simulink model "LQI_controller"  (R2024b)
settings: Solver=VariableStepAuto  StartTime=0.0  StopTime=10  RelTol=1e-3
values from neighbouring files (symbols this model uses):
  K = -F(1:2)    [State_Space_Controller.m]
  N = -F(3)    [State_Space_Controller.m]
  Ts = 0.01    [Controller.m]    (also in Controller2.m; Controller_motor_only.m; State_Space_Controller.m; dist_translate.m)
undefined symbols (not defined in the file or in its folder): dspblkCoreblockFVToolHelper, gcbh
libraries: cstblocks x1
settings Model: Creator=ethan  LastModifiedBy=ethan

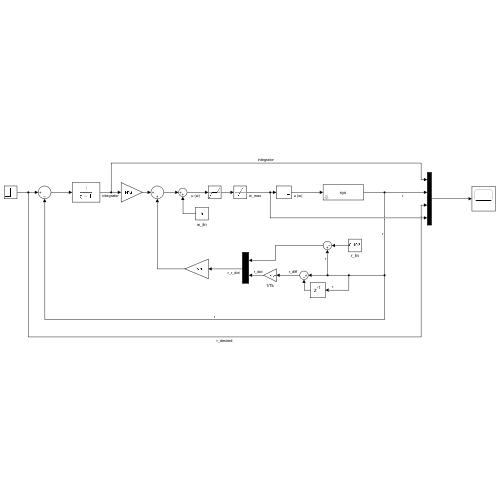
[thumbnail: Simulink's stored preview of the top-level diagram]
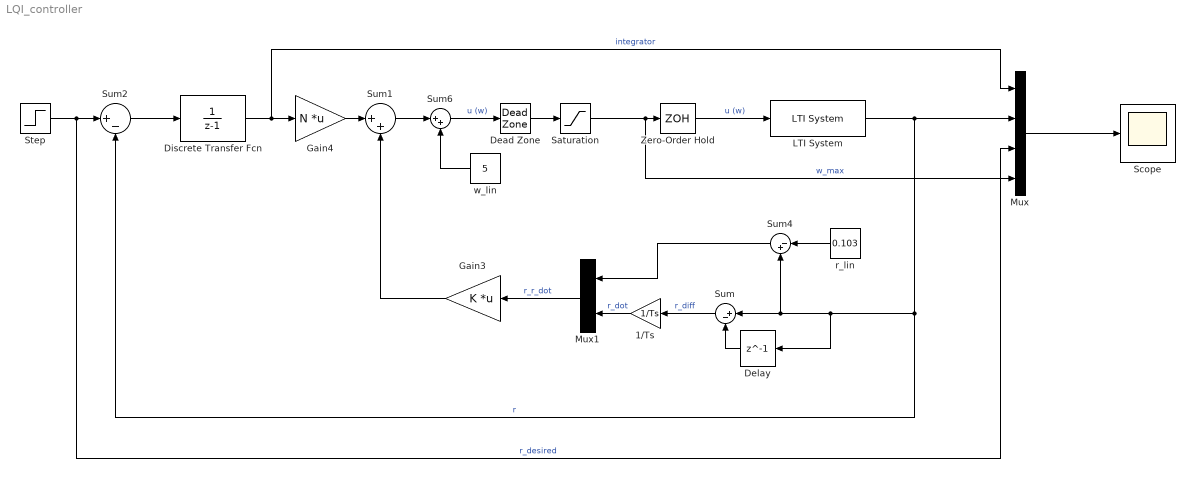
== system LQI_controller ==
  1/Ts : Gain  Gain=1/Ts
  Dead Zone : DeadZone  LowerValue=-1.75*1.811  UpperValue=1.7*1.811
  Delay : Delay  DelayLength=1  InputProcessing=Columns as channels (frame based)
  Discrete Transfer Fcn : DiscreteTransferFcn  LoadFcn=dspblkCoreblockFVToolHelper(gcbh,'load');  Denominator=[1 -1]
      settings: CopyFcn=dspblkCoreblockFVToolHelper(gcbh,'copy');  DeleteFcn=dspblkCoreblockFVToolHelper(gcbh,'close');  ModelCloseFcn=dspblkCoreblockFVToolHelper(gcbh,'close');  PreSaveFcn=dspblkCoreblockFVToolHelper(gcbh,'presave');  PostSaveFcn=dspblkCoreblockFVToolHelper(gcbh,'postsave');  CloseFcn=dspblkCoreblockFVToolHelper(gcbh,'close');
  Gain3 : Gain  Gain=K  Multiplication=Matrix(K*u)
  Gain4 : Gain  Gain=N  Multiplication=Matrix(K*u)
  LTI System : cstblocks/LTI System  sys=sys  IC=[]  PadeOrder=0
  Mux : Mux
  Mux1 : Mux  Inputs=2
  Saturation : Saturate  UpperLimit=8.30*1.811  LowerLimit=-8.42*1.811
  Scope : Scope
  Step : Step  After=0.13  SampleTime=0
  Sum : Sum  Inputs=|+-
  Sum1 : Sum  Inputs=|++
  Sum2 : Sum  Inputs=|+-
  Sum4 : Sum  Inputs=|-+
  Sum6 : Sum  Inputs=|++
  Zero-Order Hold : ZeroOrderHold  SampleTime=0.01
  r_lin : Constant  Value=0.103
  w_lin : Constant  Value=5
  wires:
  Mux/1 -> Scope/1
  Gain3/1 -> Sum1/2
  Gain4/1 -> Sum1/1
  Step/1 -> Sum2/1, Mux/3  "r_desired"
  Dead Zone/1 -> Saturation/1
  Saturation/1 -> Mux/4, Zero-Order Hold/1  "w_max"
  Sum2/1 -> Discrete Transfer Fcn/1
  Discrete Transfer Fcn/1 -> Gain4/1, Mux/1  "integrator"
  Zero-Order Hold/1 -> LTI System/1  "u (w)"
  LTI System/1 -> Mux/2, Sum2/2, Delay/1, Sum/1, Sum4/2  "r"
  1/Ts/1 -> Mux1/2  "r_dot"
  Mux1/1 -> Gain3/1  "r_r_dot"
  Sum/1 -> 1/Ts/1  "r_diff"
  Sum4/1 -> Mux1/1
  r_lin/1 -> Sum4/1
  Delay/1 -> Sum/2
  Sum1/1 -> Sum6/1
  Sum6/1 -> Dead Zone/1  "u (w)"
  w_lin/1 -> Sum6/2
